simulink subsystem "MCD"  (R2024b)
settings: Solver=VariableStepAuto  StartTime=0.0  StopTime=10.0  RelTol=1e-3
settings Model: Creator=Chenfu  LastModifiedBy=Chenfu

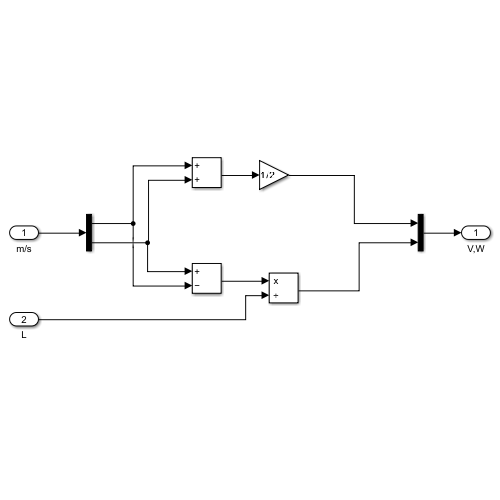
[thumbnail: Simulink's stored preview of the top-level diagram]
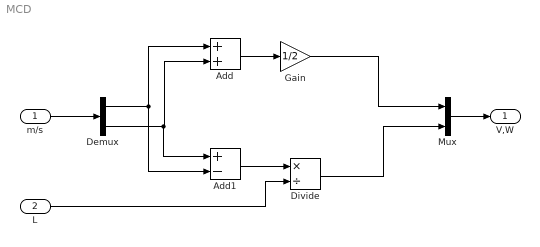
== system MCD ==
  m/s : Inport
  L : Inport  Port=2
  Add : Sum
  Add1 : Sum  Inputs=+-
  Demux : Demux  Outputs=2
  Divide : Product  Inputs=*/
  Gain : Gain  Gain=1/2
  Mux : Mux  Inputs=2
  V,W : Outport
  wires:
  Mux/1 -> V,W/1
  m/s/1 -> Demux/1
  Gain/1 -> Mux/1
  Add/1 -> Gain/1
  Demux/1 -> Add1/2, Add/1
  Demux/2 -> Add1/1, Add/2
  Add1/1 -> Divide/1
  Divide/1 -> Mux/2
  L/1 -> Divide/2
